simulink library "findClosestPathParameter_ul"  (R2020a)
settings: Solver=VariableStepAuto  StartTime=0.0  StopTime=10.0  RelTol=1e-3
libraries: calcNormalizedPathCoord_ul x1
settings Model: Creator=Ayaz  LastModifiedBy=Ayaz

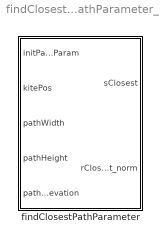
== system findClosestPathParameter_ul ==
  findClosestPathParameter : Subsystem

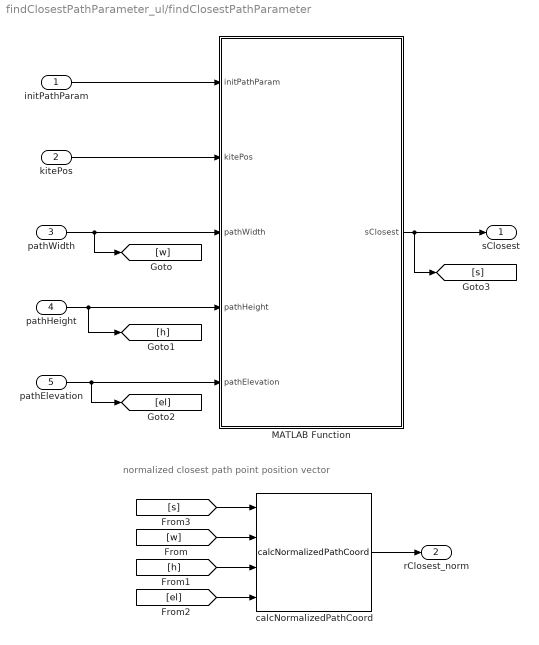
== system findClosestPathParameter_ul/findClosestPathParameter ==
  note: normalized closest path point position vector
  initPathParam : Inport
  kitePos : Inport  Port=2
  pathWidth : Inport  Port=3
  pathHeight : Inport  Port=4
  pathElevation : Inport  Port=5
  MATLAB Function : MATLAB Function  TreatAsAtomicUnit=on
  calcNormalizedPathCoord : calcNormalizedPathCoord_ul/calcNormalizedPathCoord  SystemSampleTime=-1  Latency=0  AutoFrameSizeCalculation=off
  sClosest : Outport
  rClosest_norm : Outport  Port=2
  wires:
  initPathParam/1 -> MATLAB Function/1(initPathParam)
  kitePos/1 -> MATLAB Function/2(kitePos)
  pathElevation/1 -> MATLAB Function/5(pathElevation), [el]
  pathHeight/1 -> [h], MATLAB Function/4(pathHeight)
  pathWidth/1 -> MATLAB Function/3(pathWidth), [w]
  MATLAB Function/1(sClosest) -> [s], sClosest/1
  [w] -> calcNormalizedPathCoord/2
  [h] -> calcNormalizedPathCoord/3
  [el] -> calcNormalizedPathCoord/4
  [s] -> calcNormalizedPathCoord/1
  calcNormalizedPathCoord/1 -> rClosest_norm/1

== matlab function findClosestPathParameter_ul/findClosestPathParameter/MATLAB Function ==
  data: initPathParam input; kitePos input; sClosest output; pathWidth input; pathHeight input; pathElevation input
function sClosest = findClosestPathParameter(initPathParam,kitePos,...
    pathWidth,pathHeight,pathElevation)

sClosest = findClosestPathParameter(initPathParam,kitePos,...
    pathWidth,pathHeight,pathElevation);

end
